simulink model "ActMod_Q2Trq"  (R2016b)
settings: configuration reference "CodeGenConfigSet" (kept outside this file)
PostLoadFcn:
  | , if any(exist('dsrtsu_mdlpostloadfcn', 'file') == [2, 3, 6]), try dsrtsu_mdlpostloadfcn('Execute', bdroot); catch fprintf('Error in PostLoadFcn (dsrtsu_mdlpostloadfcn) for model "%s":\n %s\n', bdroot, lasterr); end, end,
values from neighbouring files (symbols this model uses):
  ActMod_swtStrtQntEna_C = Calibration.Parameter    [init_ActMod_Q2Trq.m]    (also in init_ActMod_Q2Trq_SIL.m = Simulink.Parameter)
undefined symbols (not defined in the file or in its folder): EngState_conv, Switch_conv
settings Model: DSRTSU_INTERNAL_RTI_VER=480  DSRTSU_INTERNAL_RTI_TYPE=rti1104  Creator=Administrator  LastModifiedBy=Administrator
settings ConfigSetRef: SourceLocation=Base Workspace

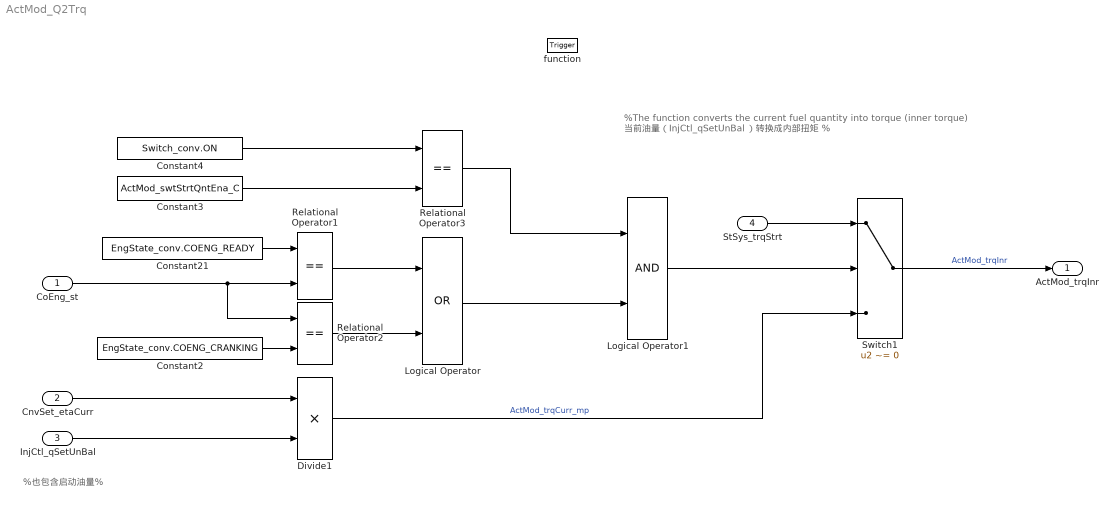
== system ActMod_Q2Trq ==
  note: %也包含启动油量%
  note: %The function converts the current fuel quantity into torque (inner torque)
      | 当前油量（InjCtl_qSetUnBal ）转换成内部扭矩 %
  CoEng_st : Inport  Description=Engine coordinator state  OutDataTypeStr=Enum: EngState_conv
  CnvSet_etaCurr : Inport  Tag=Nm/(mg/hub)  Description=Current conversion efficiency  Port=2  OutMin=-255  OutMax=255  OutDataTypeStr=TrqEta_Nm_mg_hub
  InjCtl_qSetUnBal : Inport  Tag=mg/hub  Description=Current injection quantity  Port=3  OutMin=-319  OutMax=319  OutDataTypeStr=FuelMass_mg_hub
  StSys_trqStrt : Inport  Tag=Nm  Description=Engine starting torque  Port=4  OutMin=-3000  OutMax=3000  OutDataTypeStr=Trq_Nm
  function : TriggerPort  TriggerType=function-call  VariantControl=Variant
  Constant2 : Constant  Value=EngState_conv.COENG_CRANKING  OutDataTypeStr=Inherit: Inherit via back propagation
  Constant21 : Constant  Value=EngState_conv.COENG_READY  OutDataTypeStr=Inherit: Inherit via back propagation
  Constant3 : Constant  Value=ActMod_swtStrtQntEna_C
  Constant4 : Constant  Value=Switch_conv.ON  OutDataTypeStr=Inherit: Inherit via back propagation
  Divide1 : Product  Inputs=**  OutDataTypeStr=Inherit: Inherit via back propagation  SaturateOnIntegerOverflow=on
  Logical Operator : Logic  Operator=OR  OutDataTypeStr=boolean
  Logical Operator1 : Logic  OutDataTypeStr=boolean
  Relational Operator1 : RelationalOperator  Operator===  OutDataTypeStr=boolean  RndMeth=Simplest  InputSameDT=on
  Relational Operator2 : RelationalOperator  Operator===  OutDataTypeStr=boolean  RndMeth=Simplest  InputSameDT=on
  Relational Operator3 : RelationalOperator  Operator===  OutDataTypeStr=boolean  RndMeth=Simplest  InputSameDT=on
  Switch1 : Switch  Criteria=u2 ~= 0  SaturateOnIntegerOverflow=on  InputSameDT=on
  ActMod_trqInr : Outport  Tag=Nm  Description=Current, back-calculated inner engine torque  OutMin=-3276.8  OutMax=3276.7  OutDataTypeStr=Trq_Nm
  wires:
  InjCtl_qSetUnBal/1 -> Divide1/2
  CnvSet_etaCurr/1 -> Divide1/1
  Logical Operator/1 -> Logical Operator1/2
  StSys_trqStrt/1 -> Switch1/1
  Divide1/1 -> Switch1/3  "ActMod_trqCurr_mp"
  Constant4/1 -> Relational Operator3/1
  Relational Operator3/1 -> Logical Operator1/1
  Constant3/1 -> Relational Operator3/2
  Relational Operator1/1 -> Logical Operator/1
  Constant21/1 -> Relational Operator1/1
  Constant2/1 -> Relational Operator2/2
  CoEng_st/1 -> Relational Operator2/1, Relational Operator1/2
  Relational Operator2/1 -> Logical Operator/2
  Switch1/1 -> ActMod_trqInr/1  "ActMod_trqInr"
  Logical Operator1/1 -> Switch1/2
